simulink model "LabFabSim2022a__10_6_2023"  (R2022a)
settings: Solver=VariableStepAuto  StartTime=0.0  StopTime=400  RelTol=1e-3  EnableMultiTasking=on
model workspace (MAT data in the model file):
  JsonData : timetable (value not decoded)
  M : Simulink.Parameter (value not decoded)
  ROS_trigger = 0
  SL_ROS_VariableLengthArrays_MaxSizes : object (value not decoded)
undefined symbols (not defined in the file): DOS, DOSinitGen, DTP, DTPGen, DTPInitGen, EmptyLocFound, InitCobot, InitCobotReturn, InitializeSLD, InitLEGO, InitVGRproc2, m, MC, MCGen, MCInitGen, MO, MOGen, MOInitGen, n, NetScan, NetScanInitGen, OrderGen, Spying, SpyingInitGen, WS, WSGen, WSInitGen
libraries: sldelib x1
(part 4 of 4)

== system LabFabSim2022a__10_6_2023/MaliciousControl (MC)/Subsystem1 ==
  Constant : Constant
  Out1 : Outport
  wires:
  Constant/1 -> Out1/1

== system LabFabSim2022a__10_6_2023/MaliciousOperation (MO)/InitMaliciousOperation ==
  note: On Entry: Generate 1 Malicious Operation attack entities
  Entity Generator1 : EntityGenerator  InputPortMessageModes=m  OutputPortMessageModes=m  GenerationMethod=Event-based  Period=inf  AttributeName=data  EntityType=Structured  EntityTypeName=InitMO
      settings: InputPortMap=u0
  Entity Terminator2 : EntityTerminator  InputPortMessageModes=m  EntryAction=MOGen();  NumberEntitiesArrived=on
      settings: OutputPortMap=o0
  Simulink Function2 : Subsystem  TreatAsAtomicUnit=on
  Subsystem2 : Subsystem
  Out1 : Outport
  wires:
  Subsystem2/1(Out1) -> Simulink Function2/1(In1)
  Simulink Function2/1(Out1) -> Entity Generator1/1
  Entity Terminator2/1 -> Out1/1
  Entity Generator1/1 -> Entity Terminator2/1

== system LabFabSim2022a__10_6_2023/MaliciousOperation (MO)/Malicious Operation ==
  MO : TriggerPort  TriggerType=function-call  IsSimulinkFunction=on  FunctionName=MO  VariantControl=(inherit)
  Message Send : Send  OutputPortMessageModes=m
  u : ArgIn  DisableCoverage=on  ArgumentName=u
  Out1 : Outport
  wires:
  u/1 -> Message Send/1
  Message Send/1 -> Out1/1

== system LabFabSim2022a__10_6_2023/MaliciousOperation (MO)/Simulink Function1 ==
  In1 : Inport
  MOGen : TriggerPort  TriggerType=function-call  IsSimulinkFunction=on  FunctionName=MOGen  VariantControl=(inherit)
  Message Send : Send  OutputPortMessageModes=m
  Out1 : Outport
  wires:
  Message Send/1 -> Out1/1
  In1/1 -> Message Send/1

== system LabFabSim2022a__10_6_2023/MaliciousOperation (MO)/Subsystem1 ==
  Constant : Constant
  Out1 : Outport
  wires:
  Constant/1 -> Out1/1

== system LabFabSim2022a__10_6_2023/NetworkScan/InitNetScan ==
  note: On Entry: Generate 2 NetScan attack entities
  Entity Generator1 : EntityGenerator  InputPortMessageModes=m  OutputPortMessageModes=m  GenerationMethod=Event-based  Period=inf  AttributeName=data  EntityType=Structured  EntityTypeName=InitNetScan
      settings: InputPortMap=u0
  Entity Terminator2 : EntityTerminator  InputPortMessageModes=m  EntryAction=|  NumberEntitiesArrived=on
      | for i = 1:2
      |     NetScanGen();
      | end
      settings: OutputPortMap=o0
  Simulink Function2 : Subsystem  TreatAsAtomicUnit=on
  Subsystem2 : Subsystem
  Out1 : Outport
  wires:
  Subsystem2/1(Out1) -> Simulink Function2/1(In1)
  Simulink Function2/1(Out1) -> Entity Generator1/1
  Entity Terminator2/1 -> Out1/1
  Entity Generator1/1 -> Entity Terminator2/1

== system LabFabSim2022a__10_6_2023/NetworkScan/NetScan ==
  NetScan : TriggerPort  TriggerType=function-call  IsSimulinkFunction=on  FunctionName=NetScan  VariantControl=(inherit)
  Message Send : Send  OutputPortMessageModes=m
  u : ArgIn  DisableCoverage=on  ArgumentName=u
  Out1 : Outport
  wires:
  u/1 -> Message Send/1
  Message Send/1 -> Out1/1

== system LabFabSim2022a__10_6_2023/NetworkScan/Simulink Function1 ==
  In1 : Inport
  NetScanGen : TriggerPort  TriggerType=function-call  IsSimulinkFunction=on  FunctionName=NetScanGen  VariantControl=(inherit)
  Message Send : Send  OutputPortMessageModes=m
  Out1 : Outport
  wires:
  Message Send/1 -> Out1/1
  In1/1 -> Message Send/1

== system LabFabSim2022a__10_6_2023/NetworkScan/Subsystem1 ==
  Constant : Constant
  Out1 : Outport
  wires:
  Constant/1 -> Out1/1

== system LabFabSim2022a__10_6_2023/Part Ordering/Simulink Function1 ==
  In1 : Inport
  EntityGen : TriggerPort  TriggerType=function-call  IsSimulinkFunction=on  FunctionName=EntityGen  VariantControl=(inherit)
  Message Send : Send  OutputPortMessageModes=m
  Out1 : Outport
  wires:
  Message Send/1 -> Out1/1
  In1/1 -> Message Send/1

== system LabFabSim2022a__10_6_2023/Part Ordering/Simulink Function2 ==
  In1 : Inport
  OrderGen() : TriggerPort  TriggerType=function-call  IsSimulinkFunction=on  FunctionName=OrderGen  VariantControl=(inherit)
  Message Send : Send  OutputPortMessageModes=m
  Out1 : Outport
  wires:
  Message Send/1 -> Out1/1
  In1/1 -> Message Send/1

== system LabFabSim2022a__10_6_2023/Part Ordering/Simulink Function3 ==
  ReleaseEntity : TriggerPort  TriggerType=function-call  IsSimulinkFunction=on  FunctionName=ReleaseEntity  VariantControl=(inherit)
  Constant : Constant
  Message Send : Send  OutputPortMessageModes=m
  Out1 : Outport
  wires:
  Constant/1 -> Message Send/1
  Message Send/1 -> Out1/1

== system LabFabSim2022a__10_6_2023/Part Ordering/Subsystem1 ==
  Constant : Constant
  Out1 : Outport
  wires:
  Constant/1 -> Out1/1

== system LabFabSim2022a__10_6_2023/Part Ordering/Subsystem3 ==
  Constant : Constant
  Out1 : Outport
  wires:
  Constant/1 -> Out1/1

== system LabFabSim2022a__10_6_2023/SLD (Network Scan)/Simulink Function ==
  InitVGRproc2() : TriggerPort  TriggerType=function-call  IsSimulinkFunction=on  FunctionName=InitVGRproc2  VariantControl=(inherit)
  Constant : Constant
  Message Send : Send  OutputPortMessageModes=m
  Out1 : Outport
  wires:
  Constant/1 -> Message Send/1
  Message Send/1 -> Out1/1

== system LabFabSim2022a__10_6_2023/SLD (Network Scan)/Simulink Function2 ==
  NetScan_Router : TriggerPort  TriggerType=function-call  IsSimulinkFunction=on  FunctionName=NetScan_Router  VariantControl=(inherit)
  Constant : Constant  Value=2
  Constant1 : Constant
  Switch : Switch  Threshold=2  ZeroCross=off  SaturateOnIntegerOverflow=off  InputSameDT=off
  u : ArgIn  DisableCoverage=on  ArgumentName=u
  Out1 : Outport
  wires:
  u/1 -> Switch/2
  Switch/1 -> Out1/1
  Constant1/1 -> Switch/1
  Constant/1 -> Switch/3

== system LabFabSim2022a__10_6_2023/Spying/InitSpying ==
  note: On Entry: Generate 5 Spying attack entities
  Entity Generator1 : EntityGenerator  InputPortMessageModes=m  OutputPortMessageModes=m  GenerationMethod=Event-based  Period=inf  AttributeName=data  EntityType=Structured  EntityTypeName=InitSpying
      settings: InputPortMap=u0
  Entity Terminator2 : EntityTerminator  InputPortMessageModes=m  EntryAction=|  NumberEntitiesArrived=on
      | for i = 1:5
      |     SpyingGen();
      | end
      settings: OutputPortMap=o0
  Simulink Function2 : Subsystem  TreatAsAtomicUnit=on
  Subsystem2 : Subsystem
  Out1 : Outport
  wires:
  Subsystem2/1(Out1) -> Simulink Function2/1(In1)
  Simulink Function2/1(Out1) -> Entity Generator1/1
  Entity Terminator2/1 -> Out1/1
  Entity Generator1/1 -> Entity Terminator2/1

== system LabFabSim2022a__10_6_2023/Spying/Simulink Function1 ==
  In1 : Inport
  SpyingGen : TriggerPort  TriggerType=function-call  IsSimulinkFunction=on  FunctionName=SpyingGen  VariantControl=(inherit)
  Message Send : Send  OutputPortMessageModes=m
  Out1 : Outport
  wires:
  Message Send/1 -> Out1/1
  In1/1 -> Message Send/1

== system LabFabSim2022a__10_6_2023/Spying/Spying ==
  Spying : TriggerPort  TriggerType=function-call  IsSimulinkFunction=on  FunctionName=Spying  VariantControl=(inherit)
  Message Send : Send  OutputPortMessageModes=m
  u : ArgIn  DisableCoverage=on  ArgumentName=u
  Out1 : Outport
  wires:
  u/1 -> Message Send/1
  Message Send/1 -> Out1/1

== system LabFabSim2022a__10_6_2023/Spying/Subsystem1 ==
  Constant : Constant
  Out1 : Outport
  wires:
  Constant/1 -> Out1/1

== system LabFabSim2022a__10_6_2023/VGR Moves to HBW (MO)/Simulink Function ==
  BinSupplied : TriggerPort  TriggerType=function-call  IsSimulinkFunction=on  FunctionName=BinSupplied  VariantControl=(inherit)
  Constant : Constant
  Message Send : Send  OutputPortMessageModes=m
  Out1 : Outport
  wires:
  Constant/1 -> Message Send/1
  Message Send/1 -> Out1/1

== system LabFabSim2022a__10_6_2023/VGR Moves to HBW (MO)/Simulink Function2 ==
  MO_Router : TriggerPort  TriggerType=function-call  IsSimulinkFunction=on  FunctionName=MO_Router  VariantControl=(inherit)
  Constant : Constant  Value=2
  Constant1 : Constant
  Switch : Switch  Threshold=2  ZeroCross=off  SaturateOnIntegerOverflow=off  InputSameDT=off
  u : ArgIn  DisableCoverage=on  ArgumentName=u
  Out1 : Outport
  wires:
  u/1 -> Switch/2
  Switch/1 -> Out1/1
  Constant1/1 -> Switch/1
  Constant/1 -> Switch/3

== system LabFabSim2022a__10_6_2023/VGR_Proc1 (WS & MC)/Simulink Function ==
  MPS_Initialize() : TriggerPort  TriggerType=function-call  IsSimulinkFunction=on  FunctionName=MPS_Initialize  VariantControl=(inherit)
  Constant : Constant
  Message Send : Send  OutputPortMessageModes=m
  Out1 : Outport
  wires:
  Constant/1 -> Message Send/1
  Message Send/1 -> Out1/1

== system LabFabSim2022a__10_6_2023/VGR_Proc1 (WS & MC)/Simulink Function1 ==
  MC_Router : TriggerPort  TriggerType=function-call  IsSimulinkFunction=on  FunctionName=MC_Router  VariantControl=(inherit)
  Constant : Constant  Value=2
  Constant1 : Constant
  Switch : Switch  Threshold=2  ZeroCross=off  SaturateOnIntegerOverflow=off  InputSameDT=off
  u : ArgIn  DisableCoverage=on  ArgumentName=u
  Out1 : Outport
  wires:
  u/1 -> Switch/2
  Switch/1 -> Out1/1
  Constant1/1 -> Switch/1
  Constant/1 -> Switch/3

== system LabFabSim2022a__10_6_2023/VGR_Proc1 (WS & MC)/Simulink Function2 ==
  WS_Router : TriggerPort  TriggerType=function-call  IsSimulinkFunction=on  FunctionName=WS_Router  VariantControl=(inherit)
  Constant : Constant  Value=2
  Constant1 : Constant
  Switch : Switch  Threshold=2  ZeroCross=off  SaturateOnIntegerOverflow=off  InputSameDT=off
  u : ArgIn  DisableCoverage=on  ArgumentName=u
  Out1 : Outport
  wires:
  u/1 -> Switch/2
  Switch/1 -> Out1/1
  Constant1/1 -> Switch/1
  Constant/1 -> Switch/3

== system LabFabSim2022a__10_6_2023/VGR_Proc2 (Spying)/Simulink Function ==
  InitCobot() : TriggerPort  TriggerType=function-call  IsSimulinkFunction=on  FunctionName=InitCobot  VariantControl=(inherit)
  Constant : Constant
  Message Send : Send  OutputPortMessageModes=m
  Out1 : Outport
  wires:
  Constant/1 -> Message Send/1
  Message Send/1 -> Out1/1

== system LabFabSim2022a__10_6_2023/VGR_Proc2 (Spying)/Simulink Function2 ==
  Spying_Router : TriggerPort  TriggerType=function-call  IsSimulinkFunction=on  FunctionName=Spying_Router  VariantControl=(inherit)
  Constant : Constant  Value=2
  Constant1 : Constant
  Switch : Switch  Threshold=2  ZeroCross=off  SaturateOnIntegerOverflow=off  InputSameDT=off
  u : ArgIn  DisableCoverage=on  ArgumentName=u
  Out1 : Outport
  wires:
  u/1 -> Switch/2
  Switch/1 -> Out1/1
  Constant1/1 -> Switch/1
  Constant/1 -> Switch/3

== system LabFabSim2022a__10_6_2023/VGR_Proc3 (Ramp)/Simulink Function ==
  EmptyLocFound() : TriggerPort  TriggerType=function-call  IsSimulinkFunction=on  FunctionName=EmptyLocFound  VariantControl=(inherit)
  Constant : Constant
  Message Send : Send  OutputPortMessageModes=m
  Out1 : Outport
  wires:
  Constant/1 -> Message Send/1
  Message Send/1 -> Out1/1

== system LabFabSim2022a__10_6_2023/WrongSetup (WS)/InitWrongSetup ==
  note: On Entry: Generate 1 Wrong Setup attack entities
  Entity Generator1 : EntityGenerator  InputPortMessageModes=m  OutputPortMessageModes=m  GenerationMethod=Event-based  Period=inf  AttributeName=data  EntityType=Structured  EntityTypeName=InitWS
      settings: InputPortMap=u0
  Entity Terminator2 : EntityTerminator  InputPortMessageModes=m  EntryAction=WSGen();  NumberEntitiesArrived=on
      settings: OutputPortMap=o0
  Simulink Function2 : Subsystem  TreatAsAtomicUnit=on
  Subsystem2 : Subsystem
  Out1 : Outport
  wires:
  Subsystem2/1(Out1) -> Simulink Function2/1(In1)
  Simulink Function2/1(Out1) -> Entity Generator1/1
  Entity Terminator2/1 -> Out1/1
  Entity Generator1/1 -> Entity Terminator2/1

== system LabFabSim2022a__10_6_2023/WrongSetup (WS)/Simulink Function1 ==
  In1 : Inport
  WSGen : TriggerPort  TriggerType=function-call  IsSimulinkFunction=on  FunctionName=WSGen  VariantControl=(inherit)
  Message Send : Send  OutputPortMessageModes=m
  Out1 : Outport
  wires:
  Message Send/1 -> Out1/1
  In1/1 -> Message Send/1

== system LabFabSim2022a__10_6_2023/WrongSetup (WS)/Subsystem1 ==
  Constant : Constant
  Out1 : Outport
  wires:
  Constant/1 -> Out1/1

== system LabFabSim2022a__10_6_2023/WrongSetup (WS)/Wrong Setup ==
  WS : TriggerPort  TriggerType=function-call  IsSimulinkFunction=on  FunctionName=WS  VariantControl=(inherit)
  Message Send : Send  OutputPortMessageModes=m
  u : ArgIn  DisableCoverage=on  ArgumentName=u
  Out1 : Outport
  wires:
  u/1 -> Message Send/1
  Message Send/1 -> Out1/1

== system LabFabSim2022a__10_6_2023/DOS/InitDOS/Simulink Function2 ==
  In1 : Inport
  DOSinitGen : TriggerPort  TriggerType=function-call  IsSimulinkFunction=on  FunctionName=DOSinitGen  VariantControl=(inherit)
  Message Send : Send  OutputPortMessageModes=m
  Out1 : Outport
  wires:
  Message Send/1 -> Out1/1
  In1/1 -> Message Send/1

== system LabFabSim2022a__10_6_2023/DOS/InitDOS/Subsystem2 ==
  Constant : Constant
  Out1 : Outport
  wires:
  Constant/1 -> Out1/1

== system LabFabSim2022a__10_6_2023/DataTypesProbing (DTP)/InitDataTypesProbing/Simulink Function2 ==
  In1 : Inport
  DTPInitGen : TriggerPort  TriggerType=function-call  IsSimulinkFunction=on  FunctionName=DTPInitGen  VariantControl=(inherit)
  Message Send : Send  OutputPortMessageModes=m
  Out1 : Outport
  wires:
  Message Send/1 -> Out1/1
  In1/1 -> Message Send/1

== system LabFabSim2022a__10_6_2023/DataTypesProbing (DTP)/InitDataTypesProbing/Subsystem2 ==
  Constant : Constant
  Out1 : Outport
  wires:
  Constant/1 -> Out1/1

== system LabFabSim2022a__10_6_2023/MaliciousControl (MC)/InitMaliciousControl/Simulink Function2 ==
  In1 : Inport
  MCInitGen : TriggerPort  TriggerType=function-call  IsSimulinkFunction=on  FunctionName=MCInitGen  VariantControl=(inherit)
  Message Send : Send  OutputPortMessageModes=m
  Out1 : Outport
  wires:
  Message Send/1 -> Out1/1
  In1/1 -> Message Send/1

== system LabFabSim2022a__10_6_2023/MaliciousControl (MC)/InitMaliciousControl/Subsystem2 ==
  Constant : Constant
  Out1 : Outport
  wires:
  Constant/1 -> Out1/1

== system LabFabSim2022a__10_6_2023/MaliciousOperation (MO)/InitMaliciousOperation/Simulink Function2 ==
  In1 : Inport
  MOInitGen : TriggerPort  TriggerType=function-call  IsSimulinkFunction=on  FunctionName=MOInitGen  VariantControl=(inherit)
  Message Send : Send  OutputPortMessageModes=m
  Out1 : Outport
  wires:
  Message Send/1 -> Out1/1
  In1/1 -> Message Send/1

== system LabFabSim2022a__10_6_2023/MaliciousOperation (MO)/InitMaliciousOperation/Subsystem2 ==
  Constant : Constant
  Out1 : Outport
  wires:
  Constant/1 -> Out1/1

== system LabFabSim2022a__10_6_2023/NetworkScan/InitNetScan/Simulink Function2 ==
  In1 : Inport
  NetScanInitGen : TriggerPort  TriggerType=function-call  IsSimulinkFunction=on  FunctionName=NetScanInitGen  VariantControl=(inherit)
  Message Send : Send  OutputPortMessageModes=m
  Out1 : Outport
  wires:
  Message Send/1 -> Out1/1
  In1/1 -> Message Send/1

== system LabFabSim2022a__10_6_2023/NetworkScan/InitNetScan/Subsystem2 ==
  Constant : Constant
  Out1 : Outport
  wires:
  Constant/1 -> Out1/1

== system LabFabSim2022a__10_6_2023/Spying/InitSpying/Simulink Function2 ==
  In1 : Inport
  SpyingInitGen : TriggerPort  TriggerType=function-call  IsSimulinkFunction=on  FunctionName=SpyingInitGen  VariantControl=(inherit)
  Message Send : Send  OutputPortMessageModes=m
  Out1 : Outport
  wires:
  Message Send/1 -> Out1/1
  In1/1 -> Message Send/1

== system LabFabSim2022a__10_6_2023/Spying/InitSpying/Subsystem2 ==
  Constant : Constant
  Out1 : Outport
  wires:
  Constant/1 -> Out1/1

== system LabFabSim2022a__10_6_2023/WrongSetup (WS)/InitWrongSetup/Simulink Function2 ==
  In1 : Inport
  WSInitGen : TriggerPort  TriggerType=function-call  IsSimulinkFunction=on  FunctionName=WSInitGen  VariantControl=(inherit)
  Message Send : Send  OutputPortMessageModes=m
  Out1 : Outport
  wires:
  Message Send/1 -> Out1/1
  In1/1 -> Message Send/1

== system LabFabSim2022a__10_6_2023/WrongSetup (WS)/InitWrongSetup/Subsystem2 ==
  Constant : Constant
  Out1 : Outport
  wires:
  Constant/1 -> Out1/1
